simulink model "Simu_Motorcycle_stability"  (R2020b)
settings: Solver=FixedStepAuto  StartTime=0.0  StopTime=inf  RelTol=1e-3  EnableMultiTasking=on
settings Model: SimulationMode=external  SILPILModeSetting=veronly  ExtModeTrigDuration=2  Creator=bkhusain  LastModifiedBy=gbellido
settings OptimizationCC: EnhancedBackFolding=on  PassReuseOutputArgsAs=Individual arguments  ZeroExternalMemoryAtStartup=off  ZeroInternalMemoryAtStartup=off  MaxStackSize=64  OptimizeBlockOrder=speed  DifferentSizesBufferReuse=on  OptimizationCustomize=off  EfficientTunableParamExpr=on
settings DebuggingCC: ParameterTunabilityLossMsg=error
settings HardwareCC: ProdBitPerPointer=32  ProdBitPerSizeT=32  ProdBitPerPtrDiffT=32  ProdLargestAtomicInteger=Long  ProdLargestAtomicFloat=Double  ProdWordSize=32  ProdHWDeviceType=ARM Compatible->ARM Cortex
settings SFSimCC: MATLABDynamicMemAlloc=off
settings RTWCC: Description=Embedded Coder  SystemTargetFile=ert.tlc  HardwareBoard=Arduino Nano 33 IoT  TemplateMakefile=ert_default_tmf  Toolchain=Arduino ARM  BuildConfiguration=Faster Runs
settings CodeAppCC: ForceParamTrailComments=on  IgnoreCustomStorageClasses=off  OperatorAnnotations=on  SimulinkDataObjDesc=on  SFDataObjDesc=on  InsertBlockDesc=on
settings ERTTargetCC: SupportContinuousTime=on  SupportVariableSizeSignals=on  ExtModeStaticAllocSize=8192

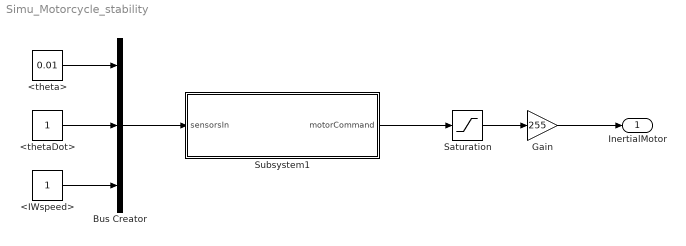
== system Simu_Motorcycle_stability ==
  <IWspeed> : Constant
  <theta> : Constant  Value=0.01
  <thetaDot> : Constant
  Bus Creator : BusCreator  Inputs=3
  Gain : Gain  Gain=255
  Saturation : Saturate  UpperLimit=1  LowerLimit=-1
  Subsystem1 : Subsystem
  InertialMotor : Outport
  wires:
  <IWspeed>/1 -> Bus Creator/3
  Subsystem1/1(motorCommand) -> Saturation/1
  <theta>/1 -> Bus Creator/1
  Gain/1 -> InertialMotor/1
  <thetaDot>/1 -> Bus Creator/2
  Bus Creator/1 -> Subsystem1/1(sensorsIn)
  Saturation/1 -> Gain/1

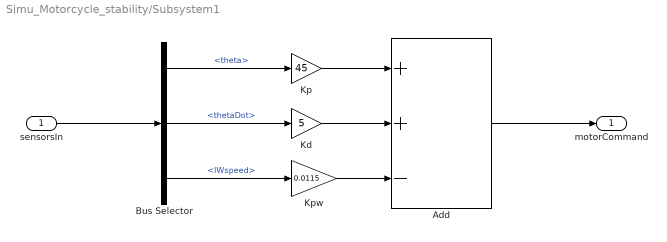
== system Simu_Motorcycle_stability/Subsystem1 ==
  sensorsIn : Inport
  Add : Sum  Inputs=++-
  Bus Selector : BusSelector  OutputSignals=theta,thetaDot,IWspeed
  Kd : Gain  Gain=5
  Kp : Gain  Gain=45
  Kpw : Gain  Gain=0.0115
  motorCommand : Outport
  wires:
  sensorsIn/1 -> Bus Selector/1
  Add/1 -> motorCommand/1
  Kpw/1 -> Add/3
  Kd/1 -> Add/2
  Kp/1 -> Add/1
  Bus Selector/1 -> Kp/1  "<theta>"
  Bus Selector/2 -> Kd/1  "<thetaDot>"
  Bus Selector/3 -> Kpw/1  "<IWspeed>"
